simulink model "EV_PV_Charging"  (R2025a)
settings: Solver=ode3  StartTime=0.0  StopTime=1  RelTol=1e-3
PreLoadFcn:
  | %% Parameter file: OBC_4_data.m
  | 
  | %% Model Parameters
  | Ts_Power= 50e-9;        % SPS Model sample time (s)
  | Co=150e-6;              % Output filter (F)
  | Ron_FET=50e-3;          % FET resistance (ohms)
  | Ron_Diode=50e-3;        % FET resistance (ohms)
  | Vf=0.6;                 % Diode forward voltage (V)
  | %
  | %% PFC Data
  | Vnom_ac= 240;           % Nominal Ac voltage (V)
  | Fnom= 60;               % System frequency (Hz)
  | L_PFC= 600e-6;          % PFC Inductance (H)
  | RL_PFC= 20e-3;          % Inductance resistance (Ohm)
  | C_PFC= 2600e-6;         % Capacitance (F)
  | 
  | %% PFC Control System Parameters
  | Ts_Control= 10e-6;      % Control system time (s)
  | Fsw= 100e3;             % PWM Switching frequency (Hz)
  | DT_PFC=400e-9;
  | %
  | % Current Regulator (PR):
  | Kp_I= 0.06;             % Proportional gain
  | Kr_I= 2.5;              % Resonant gain
  | Zeta_I=0.2;             % Damping coefficient
  | Fr_I=Fnom*2;            % Resonant frequency (Hz)
  | %
  | % Voltage Regulator (PI):
  | Kp_V= 0.25;             % Proportional gain
  | Ki_V= 80;               % Integral gain
  | Limit_V= 100;           % Output limit
  | %
  | %% LLC Data
  | Vdc_in=400;             % DC input voltage (V)
  | Vo_nom=400;             % DC nominal output voltage (V)
  | Po_nom=7.2e3;           % Nominal output power (W)
  | Lr=25e-6;               % Transformer leakage inductance (Resonant inductance in Henry)
  | Lm=150e-6;              % Magnetization inductance (H)
  | Cr=75e-9;               % Resonant capacitor (F)
  | Np=10; Ns=12; N=Np/Ns;  % Transformer ratio
  | %
  | %% LLC Control System Parameters
  | DT_LLC=400e-9;
  | Ts_Control=10e-6;
  | % Voltage Regulator (PI):
  | Kp_LLC= 100/4;          % Proportional gain
  | Ki_LLC= 150e3;          % Integral gain
  | fs_LCC_min= 120e3;      % Minimum switching frequency (Hz)
  | fs_LCC_max= 300e3;      % Maximum switching frequency (Hz)
  | Vref_LCC_min= 275;      % Minimum voltage setpoint (V)
  | Vref_LCC_max= 450;      % Maximum voltage setpoint (V)
  | %
  | %%
  | % Resonant tank data
  | Ro=Vo_nom^2/Po_nom      % LLC output load (Ohm)
  | Rac=(8/pi^2)*N^2*Ro     % Equivalent pprimary AC resistance (Ohm)
  | Q=sqrt(Lr/Cr)/Rac       % Quality factor
  | fr=1/(2*pi*sqrt(Lr*Cr)) % Resonant frequency (Hz)
  | m=(Lr+Lm)/Lr            % Ratio of total primary reactance to resonant inductance (Lr)
  | %%
InitFcn:
  | %% Parameter file: OBC_4_data.m
  | 
  | %% Model Parameters
  | Ts_Power= 50e-9;        % SPS Model sample time (s)
  | Co=150e-6;              % Output filter (F)
  | Ron_FET=50e-3;          % FET resistance (ohms)
  | Ron_Diode=50e-3;        % FET resistance (ohms)
  | Vf=0.6;                 % Diode forward voltage (V)
  | %
  | %% PFC Data
  | Vnom_ac= 240;           % Nominal Ac voltage (V)
  | Fnom= 60;               % System frequency (Hz)
  | L_PFC= 600e-6;          % PFC Inductance (H)
  | RL_PFC= 20e-3;          % Inductance resistance (Ohm)
  | C_PFC= 2600e-6;         % Capacitance (F)
  | 
  | %% PFC Control System Parameters
  | Ts_Control= 10e-6;      % Control system time (s)
  | Fsw= 100e3;             % PWM Switching frequency (Hz)
  | DT_PFC=400e-9;
  | %
  | % Current Regulator (PR):
  | Kp_I= 0.06;             % Proportional gain
  | Kr_I= 2.5;              % Resonant gain
  | Zeta_I=0.2;             % Damping coefficient
  | Fr_I=Fnom*2;            % Resonant frequency (Hz)
  | %
  | % Voltage Regulator (PI):
  | Kp_V= 0.25;             % Proportional gain
  | Ki_V= 80;               % Integral gain
  | Limit_V= 100;           % Output limit
  | %
  | %% LLC Data
  | Vdc_in=400;             % DC input voltage (V)
  | Vo_nom=400;             % DC nominal output voltage (V)
  | Po_nom=7.2e3;           % Nominal output power (W)
  | Lr=25e-6;               % Transformer leakage inductance (Resonant inductance in Henry)
  | Lm=150e-6;              % Magnetization inductance (H)
  | Cr=75e-9;               % Resonant capacitor (F)
  | Np=10; Ns=12; N=Np/Ns;  % Transformer ratio
  | %
  | %% LLC Control System Parameters
  | DT_LLC=400e-9;
  | Ts_Control=10e-6;
  | % Voltage Regulator (PI):
  | Kp_LLC= 100/4;          % Proportional gain
  | Ki_LLC= 150e3;          % Integral gain
  | fs_LCC_min= 120e3;      % Minimum switching frequency (Hz)
  | fs_LCC_max= 300e3;      % Maximum switching frequency (Hz)
  | Vref_LCC_min= 275;      % Minimum voltage setpoint (V)
  | Vref_LCC_max= 450;      % Maximum voltage setpoint (V)
  | %
  | %%
  | % Resonant tank data
  | Ro=Vo_nom^2/Po_nom      % LLC output load (Ohm)
  | Rac=(8/pi^2)*N^2*Ro     % Equivalent pprimary AC resistance (Ohm)
  | Q=sqrt(Lr/Cr)/Rac       % Quality factor
  | fr=1/(2*pi*sqrt(Lr*Cr)) % Resonant frequency (Hz)
  | m=(Lr+Lm)/Lr            % Ratio of total primary reactance to resonant inductance (Lr)
  | %%
undefined symbols (not defined in the file or in its folder): D1, Delta, DiscIntNeverNeededParam
libraries: spsSeriesRLCBranchLib x11, spsDiodeLib x7, spsMeanLib x6, MyLibrary x6, spsCurrentMeasurementLib x5, spsVoltageMeasurementLib x5, spsFourierLib x4, spsThreePhaseTransformerTwoWindingsLib x3, spsOnDelayLib x3, spsDistributedParametersLineLib x2, spsThreePhaseParallelRLCLoadLib x2, spsPWMGeneratorDCDCLib x2
(part 1 of 4)
settings Model: SimulationMode=accelerator  Creator=The MathWorks, Inc.  LastModifiedBy=changhong
settings SolverCC: AlgebraicLoopSolver=TrustRegion
settings DataIOCC: LimitDataPoints=on  SaveFormat=Array  SignalLogging=off  DSMLogging=off  ReturnWorkspaceOutputs=off
settings OptimizationCC: ExpressionDepthLimit=2147483647.0  EfficientMapNaN2IntZero=off  LifeSpan=inf
settings DebuggingCC: UnderspecifiedInitializationDetection=Classic  MergeDetectMultiDrivingBlocksExec=none  SolverPrmCheckMsg=warning  FcnCallInpInsideContextMsg=warning  UnconnectedInputMsg=warning  UnconnectedOutputMsg=warning  UnconnectedLineMsg=warning  StateNameClashWarn=warning  SubsystemReferenceDiagnosticForUnitTest=warning  SFUnexpectedBacktrackingDiag=warning  SFNoUnconditionalDefaultTransitionDiag=warning  SFExecutionAtInitializationDiag=none  ArithmeticOperatorsInVariantConditions=warning
settings HardwareCC: ProdBitPerPointer=32.0  ProdBitPerSizeT=32.0  ProdBitPerPtrDiffT=32.0  ProdLargestAtomicFloat=None  ProdIntDivRoundTo=Undefined  ProdEndianess=Unspecified  ProdWordSize=32.0  ProdHWDeviceType=32-bit Generic  TargetBitPerLong=64.0  TargetBitPerPointer=64.0  TargetBitPerSizeT=64.0  TargetBitPerPtrDiffT=64.0  TargetLongLongMode=on  TargetIntDivRoundTo=Zero  TargetEndianess=LittleEndian  TargetWordSize=64.0  TargetHWDeviceType=MATLAB Host  ProdEqTarget=off
settings ModelReferenceCC: EnableRefExpFcnMdlSchedulingChecks=on  PropagateSignalLabelsOutOfModel=off
settings SFSimCC: SimUseLocalCustomCode=off  CustomCodeUndefinedFunction=UseInterfaceOnly
settings RTWCC: GPUComputeCapability=3.5
settings CodeAppCC: MaxIdLength=128.0
settings GRTTargetCC: TargetLangStandard=C89/C90 (ANSI)  CombineOutputUpdateFcns=off  GRTInterface=on
settings ConfigComp: CovMetricSettings=dw  CovSaveCumulativeToWorkspaceVar=on  CovSaveSingleToWorkspaceVar=on  CovExternalEMLEnable=off  CovSFcnEnable=off
settings SimscapeCC: SimscapeNormalizeSystem=off

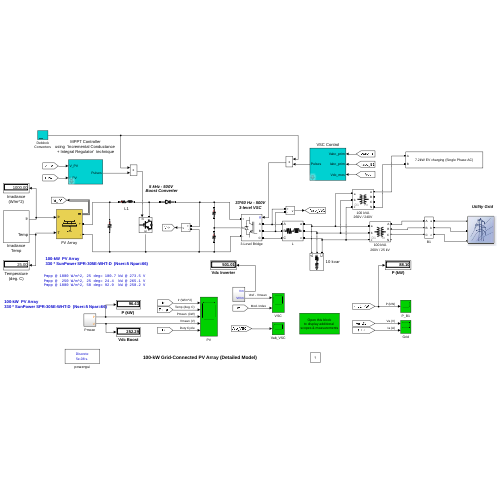
[thumbnail: Simulink's stored preview of the top-level diagram]
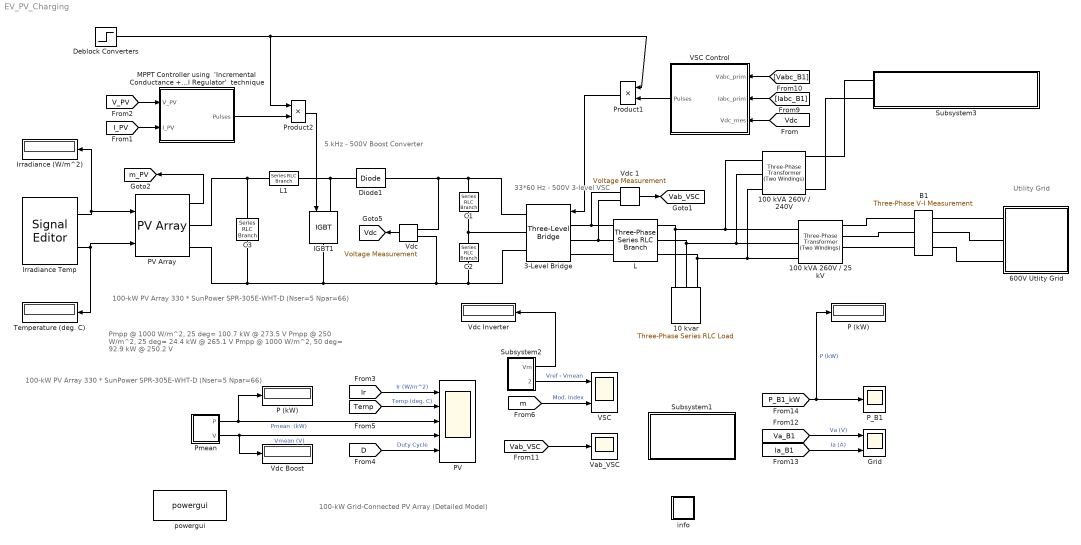
== system EV_PV_Charging ==
  note: 5 kHz - 500V
      | Boost Converter
  note: 33*60 Hz - 500V
      | 3-level VSC
  note: 100-kW Grid-Connected PV Array (Detailed Model)
  note: Utility Grid
  note: Pmpp @ 1000 W/m^2, 25 deg= 100.7 kW @ 273.5 V
      | Pmpp @  250 W/m^2, 25 deg= 24.4  kW @ 265.1 V
      | Pmpp @ 1000 W/m^2, 50 deg= 92.9  kW @ 250.2 V
  note: 100-kW  PV Array
      | 330 * SunPower SPR-305E-WHT-D  (Nser=5 Npar=66)
  note: 100-kW  PV Array
      | 330 * SunPower SPR-305E-WHT-D  (Nser=5 Npar=66)
  10 kvar : spsThreePhaseSeriesRLCLoadLib/Three-Phase Series RLC Load  LConnTagsString=A|B|C  Configuration=Y (grounded)  NominalVoltage=240  Vabc=[1e3 1e3 1e3]  Vabcp=[1e3 1e3 1e3]  NominalFrequency=60  UnbalancedPower=off  ActivePower=10e3/100  InductivePower=0  CapacitivePower=10e3  Pabc=[10e3 9e3 11e3]  QLabc=[100 90 110]  QCabc=[100 90 110]  Pabcp=[10e3 9e3 11e3]  QLabcp=[100 90 110]  QCabcp=[100 90 110]  Measurements=None  LoadType=constant Z
  100 kVA 260V / 240V : spsThreePhaseTransformerTwoWindingsLib/Three-Phase Transformer (Two Windings)  Winding1Connection=Yn  Winding2Connection=Delta (D1)  CoreType=Three single-phase transformers  SetSaturation=off  Hysteresis=off  DataFile='hysteresis'  SetInitialFlux=off  Measurements=None  UNITS=pu  NominalPower=[100e3 , 60 ]  Winding1=[ 260 , 0.001 , 0.03 ]  Winding2=[ 240*sqrt(2) , 0.001 , 0.03 ]  Rm=500  Lm=500  L0=0.5  Saturation=[ 0,0 ; 0.0024,1.2 ; 1.0,1.52 ]  InitialFluxes=[ 0.8 , -0.8 , 0.7 ]  BreakLoop=off  DiscreteSolver=Trapezoidal iterative  DataType=off  TransfoNumber=0
  100 kVA 260V / 25 kV : spsThreePhaseTransformerTwoWindingsLib/Three-Phase Transformer (Two Windings)  Winding1Connection=Yn  Winding2Connection=Delta (D1)  CoreType=Three single-phase transformers  SetSaturation=off  Hysteresis=off  DataFile='hysteresis'  SetInitialFlux=off  Measurements=None  UNITS=pu  NominalPower=[100e3 , 60 ]  Winding1=[ 25e3 , 0.001 , 0.03 ]  Winding2=[ 260 , 0.001 , 0.03 ]  Rm=500  Lm=500  L0=0.5  Saturation=[ 0,0 ; 0.0024,1.2 ; 1.0,1.52 ]  InitialFluxes=[ 0.8 , -0.8 , 0.7 ]  BreakLoop=off  DiscreteSolver=Trapezoidal iterative  DataType=off  TransfoNumber=0
  3-Level Bridge : spsThreeLevelBridgeLib/Three-Level Bridge  Arms=3  SnubberResistance=1e6  SbubberCapacitance=inf  Device=IGBT / Diodes  Ron=0.2e-3  ForwardVoltages="[  0  0 ]"  Measurements=None
      settings: AttributesFormatString=\n
  600V Utlity Grid : Subsystem
      mask Display: image('$imagefile')
  B1 : spsThreePhaseVIMeasurementLib/Three-Phase V-I Measurement  VoltageMeasurement=phase-to-ground  SetLabelV=on  LabelV=Vabc_B1  Vpu=off  VpuLL=off  CurrentMeasurement=yes  SetLabelI=on  LabelI=Iabc_B1  Ipu=off  Pbase=100e6  Vbase=500e3  OutputType=Magnitude  PhasorSimulation=off  PSBequivalent=0
  C1 : spsSeriesRLCBranchLib/Series RLC Branch  LConnTagsString=__new0  RConnTagsString=__new0  BranchType=C  Resistance=1.0  Inductance=1.0  SetiL0=off  InitialCurrent=0  Capacitance=12000e-06  Setx0=off  InitialVoltage=0  Measurements=None
  C2 : spsSeriesRLCBranchLib/Series RLC Branch  LConnTagsString=__new0  RConnTagsString=__new0  BranchType=C  Resistance=1.0  Inductance=1.0  SetiL0=off  InitialCurrent=0  Capacitance=12000e-06  Setx0=off  InitialVoltage=0  Measurements=None
  C3 : spsSeriesRLCBranchLib/Series RLC Branch  LConnTagsString=__new0  RConnTagsString=__new0  BranchType=C  Resistance=1.0  Inductance=1.0  SetiL0=off  InitialCurrent=0  Capacitance=100e-6  Setx0=off  InitialVoltage=0  Measurements=Branch voltage
  Deblock Converters : Step  Time=0.05  SampleTime=0
  Diode1 : spsDiodeLib/Diode  Ron=1e-4  Lon=0  Vf=0  IC=0  UseSnubber=off  Rs=inf  Cs=inf  Measurements=off
  Grid : Scope  NumInputPorts=2
      settings: TimeSpan=0.05  ActiveDisplayYMinimum=-5  ActiveDisplayYMaximum=5  DataLoggingDecimation=20  DataLoggingSaveFormat=Array
  IGBT1 : spsIGBTLib/IGBT  Ron=0.001  Lon=0  Vf=0  Tf=0  Tt=0  IC=0  Rs=1e5  Cs=inf  Measurements=off
  Irradiance (W/m^2) : Display
      settings: Format=bank  Decimation=1000
  Irradiance Temp : SignalEditorBlockLib/Signal Editor  FileName=PVArrayGridData.mat  ActiveScenario=Ramp_up_down_Irradiance  ActiveSignal=Temp  IsBus=off  OutputBusObjectStr=Bus: BusObject  SampleTime=0  OutputAfterFinalValue=Extrapolation  Unit=inherit  PreserveSignalName=on  ApplySigPropsToAllScenarios=on  ApplySigPropsToAllSignals=off  SignalPropertySource=Dialog parameters
  L : spsThreePhaseSeriesRLCBranchLib/Three-Phase Series RLC Branch  LConnTagsString=A|B|C  RConnTagsString=A|B|C  BranchType=RL  Resistance=500e-6*377/50/2  Inductance=500e-6/2  Capacitance=inf  Measurements=None
  L1 : spsSeriesRLCBranchLib/Series RLC Branch  LConnTagsString=__new0  RConnTagsString=__new0  BranchType=RL  Resistance=0.005  Inductance=5e-3  SetiL0=off  InitialCurrent=0  Capacitance=1e-6  Setx0=off  InitialVoltage=0  Measurements=None
  "MPPT Controller using  'Incremental Conductance + Integral Regulator'  technique " : Subsystem  mask(Boost Control - MPPT){fc=5000, T_MPPT=200e-6, Dinit=0.5}
      mask prompts: fc "PWM switching frequency (Hz)"; T_MPPT "Time window used by MPPT control (s)"; Dinit "Initial value of duty cycle"
  P (kW) : Display
      settings: Format=bank  Decimation=2000
  "P (kW) " : Display
      settings: Format=bank  Decimation=2000
  PV : Scope  NumInputPorts=5
      settings: TimeSpan=2.5  ActiveDisplayYMinimum=200  ActiveDisplayYMaximum=1000  DataLoggingDecimation=100  DataLoggingSaveFormat=Array
  PV Array : spsPVArrayLib/PV Array  Npar=66  Nser=5  PlotType=array @ 1000 W/m2 & specified temperatures  S_vec="[ 1000  250 ]"  Temp_C_vec="[0 25 50  ]"  ModuleName=SunPower SPR-305E-WHT-D  PlotWhenSelected=off  Pm=305.226  Ncell=96  Voc=64.2  Isc=5.96  Vm=54.7  Im=5.58  beta_Voc_pc=-0.2727  alpha_Isc_pc=0.061745  beta_Voc=-0.17507  alpha_Isc=0.00368  IL=5.9657  I0=6.3076e-12  nI=0.94489  Rsh=393.2054  Rs=0.37428  RobustModel=off  RobustCellTemperature=25  BAL=on  Tc=1e-6  Tfilter=5e-5
  P_B1 : Scope
      settings: TimeSpan=2.5  DataLoggingDecimation=100  DataLoggingSaveFormat=Array
  Pmean : Subsystem
  Product1 : Product  RndMeth=Zero
  Product2 : Product  RndMeth=Zero
  Subsystem1 : Subsystem
      mask Display: disp('Open this block\nto display additional \nscopes & measurements')
  Subsystem2 : Subsystem
  Subsystem3 : Subsystem
      mask Display: disp('7.2kW EV charging (Single Phase AC)');
  Temperature (deg. C) : Display
      settings: Format=bank  Decimation=1000
  VSC : Scope  NumInputPorts=2
      settings: TimeSpan=2.5  ActiveDisplayYMinimum=-5  ActiveDisplayYMaximum=5  DataLoggingDecimation=100  DataLoggingSaveFormat=Array
  VSC Control : Subsystem  mask(VSC Main Controller){nom=[ 100e3  60 ], Vnom=[ 25e3 260 ], Vnom_dc=500, RLxfo=[0.002  0.06 ], RLchoke=[2e-3  250e-6  ], K_VDCreg=[7  800], K_Ireg=[0.3 20], Ts=Ts_Control}
      mask prompts: nom "Nominal power and frequency [ Pnom(VA)  Fnom(Hz) ]:"; Vnom "Nominal primary and secondary voltages (Vrms LL) [ Vnom_prim   Vnom_sec ]:"; Vnom_dc "Nominal DC bus voltage (V):"; RLxfo "Total transformer leakage impedance (pu/Pnom) [ Rxfo  Lxf ]"; RLchoke "Choke impedance [ R(ohm) L(H) ]"; K_VDCreg "VDC regultator gains [ Kp  Ki ]:"; K_Ireg "Current regulator gains [ Kp  Ki ]:"; Ts "Sample time"
      mask init:
      | Pnom=nom(1);
      | Fnom=nom(2);
      | Vnom_prim=Vnom(1);
      | Vnom_sec=Vnom(2);
      | Zbase=Vnom_sec^2/Pnom;
      | Rtot_pu=RLxfo(1) + RLchoke(1)/Zbase;
      | Ltot_pu=RLxfo(2) + RLchoke(2)/(Zbase/(2*pi*Fnom));
      | Kp_VDCreg=K_VDCreg(1);
      | Ki_VDCreg=K_VDCreg(2);
      | Kp_Ireg=K_Ireg(1);
      | Ki_Ireg=K_Ireg(2);
      | Vdc_ref=Vnom_dc;
      | % Used to determine initial value of Boost Control (MPPT)
      | assignin('base','Vdc_ref_Inv',Vdc_ref);
  Vab_VSC : Scope
      settings: DataLoggingDecimation=10  DataLoggingSaveFormat=Array
  "Vdc " : spsVoltageMeasurementLib/Voltage Measurement  Tag=PoWeRsYsTeMmEaSuReMeNt  PhasorSimulation=off  OutputType=Magnitude  PSBequivalent=0
  Vdc 1 : spsVoltageMeasurementLib/Voltage Measurement  Tag=PoWeRsYsTeMmEaSuReMeNt  PhasorSimulation=off  OutputType=Magnitude  PSBequivalent=0
  Vdc Boost : Display
      settings: Format=bank  Decimation=2000
  Vdc Inverter : Display
      settings: Format=bank  Decimation=2000
  info : Subsystem
      settings: OpenFcn="showExample(\"simscapeelectricalsps/PVArrayGridExample\")"
      mask Display: disp('?')
  powergui : spspowerguiLib/powergui  Priority=1  SimulationMode=Discrete  SampleTime=Ts_Power  frequency=60  Iterations=50  frequencyindice=0  Pbase=100e6  ErrMax=1e-4  UnitsV=kV  UnitsW=MW  buscounter=0  FunctionMessages=off  echomessages=off  EnableUseOfTLC=off  CurrentSourceSwitches=off  DisableSnubberDevices=off  DisableRonSwitches=off  DisableVfSwitches=off  DisplayEquations=off  AutomaticDiscreteSolvers=off  SolverType=Tustin/Backward Euler (TBE)  Interpol=off  ExternalGateDelay=off  methode=off  Ts=0  x0status=blocks  SPID=off  SwTol=0  HookPort=off  NonlinearTolerance=1e-8  nMaxIteration=10  ContinueOnMaxIteration=off  RestoreLinks=warning  ResistiveCurrentMeasurement=off  Frange=[0:2:500]  Ylog=off  Xlog=on  ShowGrid=off  save=off  variable=ZData  structure=0  ZoomFFT=on  StartTime=0.0  cycles=1  DisplayStyle=1  fundamental=60  FreqAxis=off  MaxFrequency=1000  frequencyindicesteady=1  RmsSteady=1  display=off
  tag scope: Vab_VSC=global, Vdc=global, m_PV=global
  wires:
  "Vdc "/1 -> [Vdc]
  Product2/1 -> IGBT1/1
  "MPPT Controller using  'Incremental Conductance + Integral Regulator'  technique "/1(Pulses) -> Product2/2
  Deblock Converters/1 -> Product1/1, Product2/1
  [Vabc_B1] -> VSC Control/1(Vabc_prim)
  [Iabc_B1] -> VSC Control/2(Iabc_prim)
  [Vdc] -> VSC Control/3(Vdc_mes)
  VSC Control/1(Pulses) -> Product1/2
  Product1/1 -> 3-Level Bridge/1
  [I_PV] -> "MPPT Controller using  'Incremental Conductance + Integral Regulator'  technique "/2(I_PV)
  [V_PV] -> "MPPT Controller using  'Incremental Conductance + Integral Regulator'  technique "/1(V_PV)
  Pmean/1(P) -> "P (kW) "/1, PV/3  "Pmean  (kW)"
  [m] -> VSC/2  "Mod. Index"
  Vdc 1/1 -> [Vab_VSC]
  [Vab_VSC] -> Vab_VSC/1
  [Ia_B1] -> Grid/2  "Ia (A)"
  [Va_B1] -> Grid/1  "Va (V)"
  [P_B1_kW] -> P_B1/1, P (kW)/1  "P (kW)"
  Pmean/2(V) -> Vdc Boost/1, PV/4  "Vmean (V)"
  Subsystem2/2(VrVm) -> VSC/1  "Vref - Vmean"
  Subsystem2/1(Vm) -> Vdc Inverter/1
  PV Array/1 -> [m_PV]
  Irradiance Temp/1 -> PV Array/1, Irradiance (W/m^2)/1
  Irradiance Temp/2 -> PV Array/2, Temperature (deg. C)/1
  [D] -> PV/5  "Duty Cycle"
  [Temp] -> PV/2  "Temp (deg. C)"
  [Ir] -> PV/1  "Ir (W/m^2)"
  connections:
  3-Level Bridge/RConn1 -- Diode1/RConn1 -- "Vdc "/LConn1 -- C1/LConn1
  L1/RConn1 -- Diode1/LConn1 -- IGBT1/LConn1
  3-Level Bridge/RConn3 -- C2/RConn1 -- "Vdc "/LConn2 -- IGBT1/RConn1 -- PV Array/RConn2 -- C3/RConn1
  3-Level Bridge/LConn1 -- L/LConn1 -- Vdc 1/LConn1
  3-Level Bridge/LConn2 -- L/LConn2 -- Vdc 1/LConn2
  3-Level Bridge/LConn3 -- L/LConn3
  L/RConn1 -- 100 kVA 260V / 240V/RConn1 -- 100 kVA 260V / 25 kV/RConn1 -- 10 kvar/LConn1
  L/RConn2 -- 100 kVA 260V / 240V/RConn2 -- 100 kVA 260V / 25 kV/RConn2 -- 10 kvar/LConn2
  L/RConn3 -- 100 kVA 260V / 240V/RConn3 -- 100 kVA 260V / 25 kV/RConn3 -- 10 kvar/LConn3
  B1/LConn2 -- 100 kVA 260V / 25 kV/LConn2
  B1/LConn3 -- 100 kVA 260V / 25 kV/LConn3
  C2/LConn1 -- C1/RConn1 -- 3-Level Bridge/RConn2
  C3/LConn1 -- PV Array/RConn1 -- L1/LConn1
  B1/RConn2 -- 600V Utlity Grid/LConn2
  B1/RConn1 -- 600V Utlity Grid/LConn1
  B1/RConn3 -- 600V Utlity Grid/LConn3
  100 kVA 260V / 25 kV/LConn1 -- B1/LConn1
  100 kVA 260V / 240V/LConn1 -- Subsystem3/LConn1
  100 kVA 260V / 240V/LConn4 -- Subsystem3/LConn2
